simulink model "Model"  (R2022b)
settings: Solver=VariableStepAuto  StartTime=0.0  StopTime=15  RelTol=1e-3
values from neighbouring files (symbols this model uses):
  a0 = 0.5452    [MNK_New.m]
  a1 = 2.9780    (= 2.978)    [MNK_New.m]
  alpha_filt = 0.025    [MNK_New.m]
  b = 0.9827    [MNK_New.m]
  W_Pid = tf_p + tf_i + tf_D    [Pid_W_function.m]
libraries: slpidlib x1
settings Model: Creator=ilya  LastModifiedBy=ilya

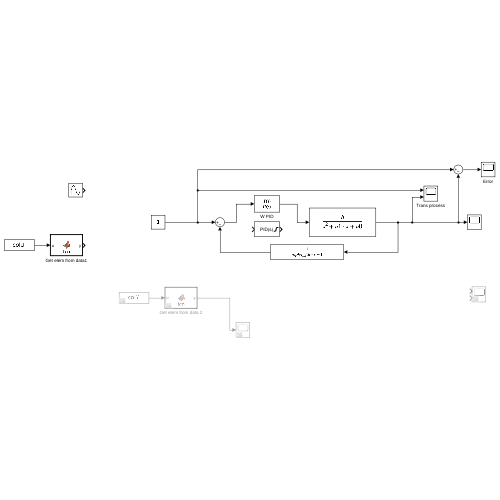
[thumbnail: Simulink's stored preview of the top-level diagram]
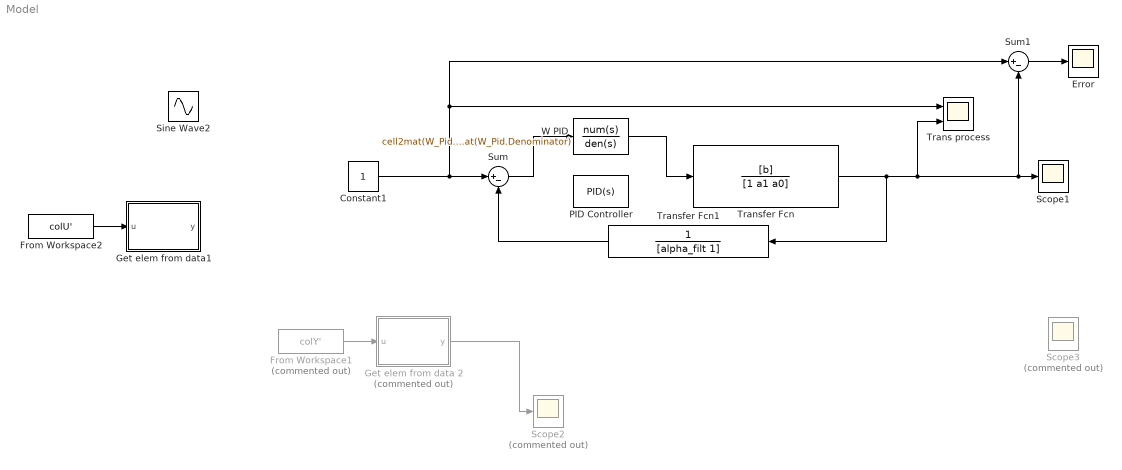
== system Model ==
  Constant1 : Constant
  Error : Scope
  From Workspace1 : FromWorkspace  Commented=on  VariableName=colY'  SampleTime=0.025
  From Workspace2 : FromWorkspace  VariableName=colU'  OutDataTypeStr=double  SampleTime=0.025
  Get elem from data 2 : MATLAB Function  Commented=on  TreatAsAtomicUnit=on
  Get elem from data1 : MATLAB Function  TreatAsAtomicUnit=on
  PID Controller : slpidlib/PID Controller  Controller=PID  Form=Parallel  TimeDomain=Continuous-time  UseExternalTs=off  SampleTime=-1  IntegratorMethod=Forward Euler  FilterMethod=Forward Euler  ControllerParametersSource=internal  P=6.68519117883399  I=3.41356175675233  UseKiTs=off  D=1.64826423496531  N=4.79339804476038  UseFilter=on  TunerSelectOption=Transfer Function Based (PID Tuner App)  InitialConditionSource=internal  InitialConditionForIntegrator=1  InitialConditionForFilter=0  DifferentiatorICPrevScaledInput=0  ExternalReset=none  TrackingMode=off  Kt=1  LimitOutput=on  SatLimitsSource=internal  UpperSaturationLimit=inf  LowerSaturationLimit=-inf  LinearizeAsGain=on  AntiWindupMode=clamping  Kb=1  LimitIntegrator=off  UpperIntegratorSaturationLimit=inf  LowerIntegratorSaturationLimit=-inf  POutMin=[]  POutMax=[]  IOutMin=[]  IOutMax=[]  DOutMin=[]  DOutMax=[]  NOutMin=[]  NOutMax=[]  SumOutMin=[]  SumOutMax=[]  SaturationOutMin=[]  SaturationOutMax=[]  PParamMin=[]  PParamMax=[]  IParamMin=[]  IParamMax=[]  DParamMin=[]  DParamMax=[]  NParamMin=[]  NParamMax=[]  KbParamMin=[]  KbParamMax=[]  KtParamMin=[]  KtParamMax=[]  KbOutMin=[]  KbOutMax=[]  KtOutMin=[]  KtOutMax=[]  IntegratorOutMin=[]  IntegratorOutMax=[]  FilterOutMin=[]  FilterOutMax=[]  SumI1OutMin=[]  SumI1OutMax=[]  SumI2OutMin=[]  SumI2OutMax=[]  SumI3OutMin=[]  SumI3OutMax=[]  SumI4OutMin=[]  SumI4OutMax=[]  SumDOutMin=[]  SumDOutMax=[]  DifferentiatorOutMin=[]  DifferentiatorOutMax=[]  FilterDiffOutCoefMin=[]  FilterDiffOutCoefMax=[]  ReciprocalOutMin=[]  ReciprocalOutMax=[]  SumDenOutMin=[]  SumDenOutMax=[]  SumNumOutMin=[]  SumNumOutMax=[]  DivideOutMin=[]  DivideOutMax=[]  UdiffTsProdOutMin=[]  UdiffTsProdOutMax=[]  NTsProdOutMin=[]  NTsProdOutMax=[]  UintegralTsProdOutMin=[]  UintegralTsProdOutMax=[]  UngainTsProdOutMin=[]  UngainTsProdOutMax=[]  ClampingZeroOutDataTypeStr=Inherit: Inherit via back propagation  ClampingZeroOutMin=[]  ClampingZeroOutMax=[]  FilterDenConstantOutDataTypeStr=Inherit: Inherit via back propagation  FilterDenConstantOutMin=[]  FilterDenConstantOutMax=[]  PCopyOutDataTypeStr=Inherit: Inherit via back propagation  PCopyOutMin=[]  PCopyOutMax=[]  NCopyOutDataTypeStr=Inherit: Inherit via back propagation  NCopyOutMin=[]  NCopyOutMax=[]  IntegratorContinuousStateAttributes=''  IntegratorStateMustResolveToSignalObject=off  IntegratorRTWStateStorageClass=Auto  FilterContinuousStateAttributes=''  FilterStateMustResolveToSignalObject=off  FilterRTWStateStorageClass=Auto  ParallelPVariant=InternalParameters  IdealPVariant=Disabled  IVariant=InternalParameters  DVariant=InternalParameters  IntegratorVariant=Continuous  SatVariant=Enabled  AWVariant=ContClampingParallel  PCopyVariant=Disabled  TRVariant=Disabled  FdbkBlocksVariant=Forward  IdealPFdbkVariant=Disabled  SatFdbkVariant=Disabled  DerivativeFilterVariant=ContFilter  NVariant=InternalParameters  NCopyVariant=Disabled  FilterICVariant=InternalICsFilter  IntegratorICVariant=InternalICs  ExternalResetVariant=Disabled  TRSumVariant=Passthrough  SumFdbkVariant=Disabled  SumVariant=Sum_PID  TsampFilterVariant=InternalTs  TsampNgainVariant=Passthrough  TsampIntegralVariant=Passthrough  ExternalSaturationOutDataTypeStr=Inherit: Same as second input
  Scope1 : Scope
  Scope2 : Scope  Commented=on
  Scope3 : Scope  Commented=on  NumInputPorts=2
  Sine Wave2 : Sin  SampleTime=0
  Sum : Sum  Inputs=|+-
  Sum1 : Sum  Inputs=|+-
  Trans process : Scope  NumInputPorts=2
  Transfer Fcn : TransferFcn  Numerator=[b]  Denominator=[1 a1 a0]
  Transfer Fcn1 : TransferFcn  Denominator=[alpha_filt 1]
  W PID : TransferFcn  Numerator=cell2mat(W_Pid.Numerator)  Denominator=cell2mat(W_Pid.Denominator)
  wires:
  Transfer Fcn/1 -> Transfer Fcn1/1, Sum1/2, Scope1/1, Trans process/2
  From Workspace1/1 -> Get elem from data 2/1(u)
  Get elem from data 2/1(y) -> Scope2/1
  Constant1/1 -> Sum1/1, Trans process/1, Sum/1
  Sum1/1 -> Error/1
  Transfer Fcn1/1 -> Sum/2
  From Workspace2/1 -> Get elem from data1/1(u)
  Sum/1 -> W PID/1
  W PID/1 -> Transfer Fcn/1

== matlab function Model/Get elem from data1 ==
  data: u input; y output
function y = fcn(u)
persistent ind;
if isempty(ind)
    ind = 0;
end

ind = ind + 1;

y = u(ind);

== matlab function Model/Get elem from data 2 ==
  data: u input; y output
function y = fcn(u)
persistent ind;
if isempty(ind)
    ind = 0;
end

ind = ind + 1;

y = u(ind);
